simulink model "SVM_Blocks"  (R2021a)
settings: Solver=ode23s  StartTime=0.0  StopTime=.02*20  MaxStep=1e-5  RelTol=1e-3
libraries: spsThreePhaseVIMeasurementLib x5, spsSVPWMGenerator2LevelLib x4, spsThreePhaseSeriesRLCBranchLib x4, spsVoltageMeasurementLib x4, spsDCVoltageSourceLib x3, spsUniversalBridgeLib x3, dsparch4 x2, spsGroundLib x2, spsRMSLib x2, spsAsynchronousMachineSIUnitsLib x1, spsabctoAlphaBetaZeroLib x1, spspowerguiLib x1
settings Model: Creator=Ahmed Mohamed  LastModifiedBy=Ahmed Mohamed
settings DataIOCC: ReturnWorkspaceOutputs=off

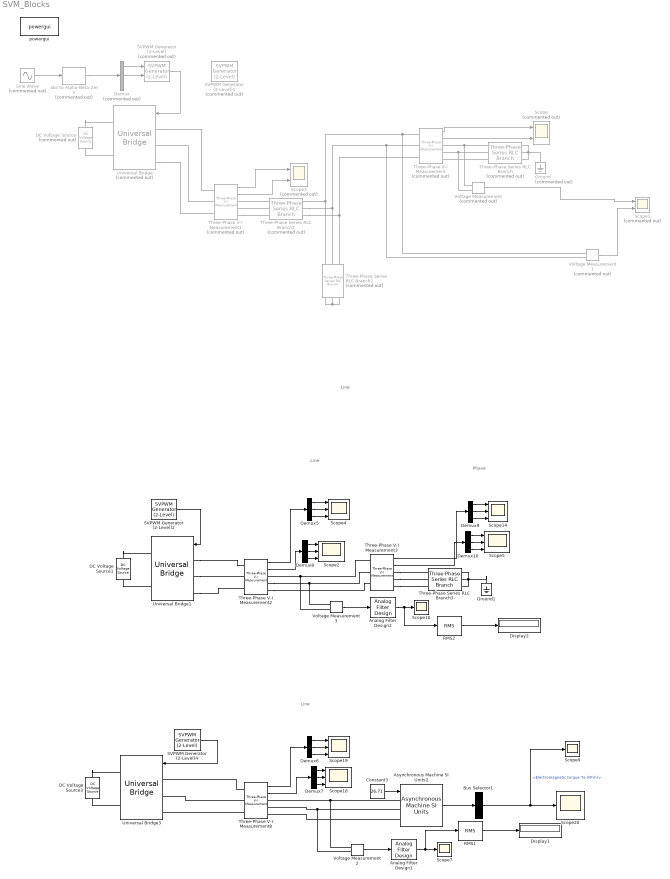
== system SVM_Blocks ==
  note: Line
  note: Phase
  note: Line
  note: Line
  Analog Filter Design1 : dsparch4/Analog Filter Design  method=Butterworth  filttype=Lowpass  N=8  Wlo=2*pi*1000  Whi=80  Rp=2  Rs=40
  Analog Filter Design2 : dsparch4/Analog Filter Design  method=Butterworth  filttype=Lowpass  N=8  Wlo=2*pi*500  Whi=80  Rp=2  Rs=40
  Asynchronous Machine SI Units2 : spsAsynchronousMachineSIUnitsLib/Asynchronous Machine SI Units  RotorType=Squirrel-cage  PresetModel="15:  5.4 HP (4KW)   400 V  50Hz 1430 RPM"  MechanicalLoad=Torque Tm  ShowDetailedParameters=on  ReferenceFrame=Rotor  Units=SI  MeasurementBus=off  NominalParameters=[4000 400 50]  VoltageRatio=1  Stator=[1.405 0.005839]  Rotor=[1.395 0.005839]  Cage1=[0.4155 0.002066]  Cage2=[0.4168 0.0003495]  Lm=0.1722  Mechanical=[0.0131 0.002985 2]  PolePairs=2  InitialConditions=[1 0 0 0 0 0 0 0]  SimulateSaturation=off  Saturation=[14.03593122, 27.81365428, 53.79336849, 72.68890987, 97.98006896, 148.6815601, 215.7428561, 302.9841135, 428.7778367 ; 230, 322, 414, 460, 506, 552, 598, 644, 690]  LoadFlowParameters=1492000  TsPowergui=0  TsBlock=-1  IterativeModel=Trapezoidal non iterative  IterativeDiscreteModel=Trapezoidal non iterative  Pmec=1.492e+006
  Bus Selector1 : BusSelector  OutputSignals=Mechanical.Electromagnetic torque Te (N*m)
  Constant3 : Constant  Value=26.71
  DC Voltage Source : spsDCVoltageSourceLib/DC Voltage Source  Commented=on  Amplitude=540  Measurements=None
  DC Voltage Source1 : spsDCVoltageSourceLib/DC Voltage Source  Amplitude=570  Measurements=None
  DC Voltage Source3 : spsDCVoltageSourceLib/DC Voltage Source  Amplitude=570  Measurements=None
  Demux : Demux  Commented=on  Outputs=3
  Demux{5..10} (6 alike) : Demux  Outputs=3
  Display1 : Display
  Display2 : Display
  Ground : spsGroundLib/Ground  Commented=on  LConnTagsString=a
  Ground1 : spsGroundLib/Ground  LConnTagsString=a
  RMS1 : spsRMSLib/RMS  TrueRMS=off  Freq=50  RMSInit=0  Ts=0
  RMS2 : spsRMSLib/RMS  TrueRMS=off  Freq=50  RMSInit=0  Ts=0
  SVPWM Generator (2-Level) : spsSVPWMGenerator2LevelLib/SVPWM Generator (2-Level)  Commented=on  InputType=alpha-beta components  SwitchingPattern=Pattern #1  Fc=5000  ParUref=[0.8 -30 50]  Ts=0
      settings: SourceProductBaseCode=PS
  SVPWM Generator (2-Level)1 : spsSVPWMGenerator2LevelLib/SVPWM Generator (2-Level)  Commented=on  InputType=Internally generated  SwitchingPattern=Pattern #2  Fc=5000  ParUref=[0.8 -30 50]  Ts=0
      settings: SourceProductBaseCode=PS
  SVPWM Generator (2-Level)2 : spsSVPWMGenerator2LevelLib/SVPWM Generator (2-Level)  InputType=Internally generated  SwitchingPattern=Pattern #1  Fc=10000  ParUref=[1 0 50]  Ts=0
      settings: SourceProductBaseCode=PS
  SVPWM Generator (2-Level)4 : spsSVPWMGenerator2LevelLib/SVPWM Generator (2-Level)  InputType=Internally generated  SwitchingPattern=Pattern #1  Fc=10000  ParUref=[1 0 50]  Ts=0
      settings: SourceProductBaseCode=PS
  Scope : Scope  Commented=on  NumInputPorts=2
  Scope1 : Scope  Commented=on  NumInputPorts=2
  Scope{7,9..10,20} (4 alike) : Scope
  Scope{2,4..5,14,18..19} (6 alike) : Scope  NumInputPorts=3
  Scope3 : Scope  Commented=on  NumInputPorts=2
  Sine Wave : Sin  Commented=on  Amplitude=.99  Frequency=2*50*pi  Phase=[0 -2*pi/3 2*pi/3]  SampleTime=0
  Three-Phase Series RLC Branch : spsThreePhaseSeriesRLCBranchLib/Three-Phase Series RLC Branch  Commented=on  LConnTagsString=A|B|C  RConnTagsString=A|B|C  BranchType=R  Resistance=10  Inductance=1e-3  Capacitance=1e-6  Measurements=None
  Three-Phase Series RLC Branch1 : spsThreePhaseSeriesRLCBranchLib/Three-Phase Series RLC Branch  Commented=on  LConnTagsString=A|B|C  RConnTagsString=A|B|C  BranchType=L  Resistance=10  Inductance=1e-3  Capacitance=1e-6  Measurements=None
  Three-Phase Series RLC Branch2 : spsThreePhaseSeriesRLCBranchLib/Three-Phase Series RLC Branch  Commented=on  LConnTagsString=A|B|C  RConnTagsString=A|B|C  BranchType=C  Resistance=10  Inductance=1e-3  Capacitance=100e-6  Measurements=None
  Three-Phase Series RLC Branch3 : spsThreePhaseSeriesRLCBranchLib/Three-Phase Series RLC Branch  LConnTagsString=A|B|C  RConnTagsString=A|B|C  BranchType=RL  Resistance=7.5*sqrt(2)  Inductance=7.5*sqrt(2)/314  Capacitance=1e-6  Measurements=None
  Three-Phase V-I Measurement : spsThreePhaseVIMeasurementLib/Three-Phase V-I Measurement  Commented=on  VoltageMeasurement=phase-to-ground  SetLabelV=off  LabelV=Vabc  Vpu=off  VpuLL=off  CurrentMeasurement=yes  SetLabelI=off  LabelI=Iabc  Ipu=off  Pbase=100e6  Vbase=500e3  OutputType=Complex  PhasorSimulation=off  PSBequivalent=0
  Three-Phase V-I Measurement1 : spsThreePhaseVIMeasurementLib/Three-Phase V-I Measurement  Commented=on  VoltageMeasurement=phase-to-phase  SetLabelV=off  LabelV=Vabc  Vpu=off  VpuLL=off  CurrentMeasurement=yes  SetLabelI=off  LabelI=Iabc  Ipu=off  Pbase=100e6  Vbase=500e3  OutputType=Complex  PhasorSimulation=off  PSBequivalent=0
  Three-Phase V-I Measurement2 : spsThreePhaseVIMeasurementLib/Three-Phase V-I Measurement  VoltageMeasurement=phase-to-phase  SetLabelV=off  LabelV=Vabc  Vpu=off  VpuLL=off  CurrentMeasurement=yes  SetLabelI=off  LabelI=Iabc  Ipu=off  Pbase=100e6  Vbase=500e3  OutputType=Complex  PhasorSimulation=off  PSBequivalent=0
  Three-Phase V-I Measurement3 : spsThreePhaseVIMeasurementLib/Three-Phase V-I Measurement  VoltageMeasurement=phase-to-ground  SetLabelV=off  LabelV=Vabc  Vpu=off  VpuLL=off  CurrentMeasurement=yes  SetLabelI=off  LabelI=Iabc  Ipu=off  Pbase=100e6  Vbase=500e3  OutputType=Complex  PhasorSimulation=off  PSBequivalent=0
  Three-Phase V-I Measurement8 : spsThreePhaseVIMeasurementLib/Three-Phase V-I Measurement  VoltageMeasurement=phase-to-phase  SetLabelV=off  LabelV=Vabc  Vpu=off  VpuLL=off  CurrentMeasurement=yes  SetLabelI=off  LabelI=Iabc  Ipu=off  Pbase=100e6  Vbase=500e3  OutputType=Complex  PhasorSimulation=off  PSBequivalent=0
  Universal Bridge : spsUniversalBridgeLib/Universal Bridge  Commented=on  Arms=3  SnubberResistance=1e5  SnubberCapacitance=inf  Device=IGBT / Diodes  Ron=1e-3  Lon=0  ForwardVoltages="[  0  0  ]"  ForwardVoltage=0  GTOparameters=[ 10e-6 , 20e-6 ]  IGBTparameters=[ 1e-6 , 2e-6 ]  Measurements=None  Measurements_2=None  converterType=Rectifier
  Universal Bridge1 : spsUniversalBridgeLib/Universal Bridge  Arms=3  SnubberResistance=1e5  SnubberCapacitance=inf  Device=IGBT / Diodes  Ron=1e-3  Lon=0  ForwardVoltages="[  0  0  ]"  ForwardVoltage=0  GTOparameters=[ 10e-6 , 20e-6 ]  IGBTparameters=[ 1e-6 , 2e-6 ]  Measurements=None  Measurements_2=None  converterType=Rectifier
  Universal Bridge3 : spsUniversalBridgeLib/Universal Bridge  Arms=3  SnubberResistance=1e5  SnubberCapacitance=inf  Device=IGBT / Diodes  Ron=1e-3  Lon=0  ForwardVoltages="[  0  0  ]"  ForwardVoltage=0  GTOparameters=[ 10e-6 , 20e-6 ]  IGBTparameters=[ 1e-6 , 2e-6 ]  Measurements=None  Measurements_2=None  converterType=Rectifier
  Voltage Measurement : spsVoltageMeasurementLib/Voltage Measurement  Commented=on  PhasorSimulation=off  OutputType=Complex  PSBequivalent=0
  Voltage Measurement1 : spsVoltageMeasurementLib/Voltage Measurement  Commented=on  PhasorSimulation=off  OutputType=Complex  PSBequivalent=0
  Voltage Measurement2 : spsVoltageMeasurementLib/Voltage Measurement  PhasorSimulation=off  OutputType=Complex  PSBequivalent=0
  Voltage Measurement3 : spsVoltageMeasurementLib/Voltage Measurement  PhasorSimulation=off  OutputType=Complex  PSBequivalent=0
  abc to Alpha-Beta-Zero : spsabctoAlphaBetaZeroLib/abc to Alpha-Beta-Zero  Commented=on
      settings: SourceProductBaseCode=PS
  powergui : spspowerguiLib/powergui  Priority=1  SimulationMode=Continuous  SampleTime=50e-6  frequency=60  Iterations=50  frequencyindice=0  Pbase=100e6  ErrMax=1e-4  UnitsV=kV  UnitsW=MW  buscounter=0  FunctionMessages=off  echomessages=off  EnableUseOfTLC=off  CurrentSourceSwitches=off  DisableSnubberDevices=off  DisableRonSwitches=off  DisableVfSwitches=off  DisplayEquations=off  AutomaticDiscreteSolvers=off  SolverType=Tustin/Backward Euler (TBE)  Interpol=off  ExternalGateDelay=off  methode=off  Ts=100  x0status=blocks  SPID=on  SwTol=0  HookPort=off  NonlinearTolerance=1e-4  nMaxIteration=100  ContinueOnMaxIteration=off  RestoreLinks=warning  ResistiveCurrentMeasurement=off  Frange=[0:2:500]  Ylog=off  Xlog=on  ShowGrid=off  save=off  variable=ZData  structure=0  ZoomFFT=off  StartTime=0.0  cycles=1  DisplayStyle=1  fundamental=60  FreqAxis=off  MaxFrequency=1000  frequencyindicesteady=1  RmsSteady=1  display=off
  wires:
  Sine Wave/1 -> abc to Alpha-Beta-Zero/1
  abc to Alpha-Beta-Zero/1 -> Demux/1
  Demux/1 -> SVPWM Generator (2-Level)/1
  Demux/2 -> SVPWM Generator (2-Level)/2
  SVPWM Generator (2-Level)/1 -> Universal Bridge/1
  Three-Phase V-I Measurement/1 -> Scope/1
  Three-Phase V-I Measurement/2 -> Scope/2
  Voltage Measurement/1 -> Scope1/1
  Three-Phase V-I Measurement1/1 -> Scope3/1
  Three-Phase V-I Measurement1/2 -> Scope3/2
  Voltage Measurement1/1 -> Scope1/2
  SVPWM Generator (2-Level)2/1 -> Universal Bridge1/1
  Demux10/1 -> Scope5/1
  Demux5/1 -> Scope4/1
  Demux5/3 -> Scope4/3
  Demux10/3 -> Scope5/3
  Demux9/3 -> Scope14/3
  Three-Phase V-I Measurement3/2 -> Demux10/1
  Three-Phase V-I Measurement3/1 -> Demux9/1
  Demux5/2 -> Scope4/2
  Demux10/2 -> Scope5/2
  Demux8/1 -> Scope2/1
  Demux9/2 -> Scope14/2
  Three-Phase V-I Measurement2/2 -> Demux8/1
  Demux8/2 -> Scope2/2
  Three-Phase V-I Measurement2/1 -> Demux5/1
  Demux9/1 -> Scope14/1
  Demux8/3 -> Scope2/3
  SVPWM Generator (2-Level)4/1 -> Universal Bridge3/1
  Three-Phase V-I Measurement8/1 -> Demux6/1
  Asynchronous Machine SI Units2/1 -> Bus Selector1/1
  Three-Phase V-I Measurement8/2 -> Demux7/1
  Bus Selector1/1 -> Scope9/1, Scope20/1  "<Electromagnetic torque Te (N*m)>"
  Demux7/3 -> Scope18/3
  Demux7/2 -> Scope18/2
  Demux6/1 -> Scope19/1
  Demux7/1 -> Scope18/1
  Demux6/3 -> Scope19/3
  Constant3/1 -> Asynchronous Machine SI Units2/1
  Demux6/2 -> Scope19/2
  RMS1/1 -> Display1/1
  Analog Filter Design1/1 -> Scope7/1, RMS1/1
  Voltage Measurement2/1 -> Analog Filter Design1/1
  Voltage Measurement3/1 -> Analog Filter Design2/1
  Analog Filter Design2/1 -> Scope10/1, RMS2/1
  RMS2/1 -> Display2/1
  connections:
  DC Voltage Source/RConn1 -- Universal Bridge/RConn1
  DC Voltage Source/LConn1 -- Universal Bridge/RConn2
  Three-Phase V-I Measurement1/LConn2 -- Universal Bridge/LConn2
  Universal Bridge/LConn1 -- Three-Phase V-I Measurement1/LConn1
  Universal Bridge/LConn3 -- Three-Phase V-I Measurement1/LConn3
  Three-Phase Series RLC Branch/LConn1 -- Voltage Measurement/LConn1 -- Three-Phase V-I Measurement/RConn1
  Three-Phase Series RLC Branch/LConn2 -- Voltage Measurement/LConn2 -- Three-Phase V-I Measurement/RConn2
  Three-Phase Series RLC Branch/LConn3 -- Three-Phase V-I Measurement/RConn3
  Three-Phase Series RLC Branch/RConn1 -- Ground/LConn1 -- Three-Phase Series RLC Branch/RConn2 -- Three-Phase Series RLC Branch/RConn3
  Three-Phase Series RLC Branch1/LConn1 -- Three-Phase V-I Measurement1/RConn1
  Three-Phase Series RLC Branch1/LConn2 -- Three-Phase V-I Measurement1/RConn2
  Three-Phase Series RLC Branch1/RConn1 -- Voltage Measurement1/LConn1 -- Three-Phase V-I Measurement/LConn1 -- Three-Phase Series RLC Branch2/LConn1
  Three-Phase Series RLC Branch1/RConn2 -- Voltage Measurement1/LConn2 -- Three-Phase V-I Measurement/LConn2 -- Three-Phase Series RLC Branch2/LConn2
  Three-Phase Series RLC Branch1/RConn3 -- Three-Phase V-I Measurement/LConn3 -- Three-Phase Series RLC Branch2/LConn3
  Three-Phase Series RLC Branch2/RConn1 -- Three-Phase Series RLC Branch2/RConn2 -- Three-Phase Series RLC Branch2/RConn3
  Three-Phase V-I Measurement1/RConn3 -- Three-Phase Series RLC Branch1/LConn3
  DC Voltage Source1/RConn1 -- Universal Bridge1/RConn1
  DC Voltage Source1/LConn1 -- Universal Bridge1/RConn2
  Three-Phase Series RLC Branch3/RConn2 -- Three-Phase Series RLC Branch3/RConn3 -- Three-Phase Series RLC Branch3/RConn1 -- Ground1/LConn1
  Three-Phase V-I Measurement3/RConn3 -- Three-Phase Series RLC Branch3/LConn3
  Three-Phase V-I Measurement3/RConn2 -- Three-Phase Series RLC Branch3/LConn2
  Three-Phase V-I Measurement2/RConn3 -- Three-Phase V-I Measurement3/LConn3
  Three-Phase V-I Measurement3/LConn1 -- Voltage Measurement3/LConn2 -- Three-Phase V-I Measurement2/RConn1
  Three-Phase V-I Measurement2/RConn2 -- Voltage Measurement3/LConn1 -- Three-Phase V-I Measurement3/LConn2
  Three-Phase V-I Measurement3/RConn1 -- Three-Phase Series RLC Branch3/LConn1
  Universal Bridge1/LConn1 -- Three-Phase V-I Measurement2/LConn1
  Universal Bridge1/LConn2 -- Three-Phase V-I Measurement2/LConn2
  Universal Bridge1/LConn3 -- Three-Phase V-I Measurement2/LConn3
  Three-Phase V-I Measurement8/LConn3 -- Universal Bridge3/LConn3
  Three-Phase V-I Measurement8/LConn1 -- Universal Bridge3/LConn1
  Three-Phase V-I Measurement8/LConn2 -- Universal Bridge3/LConn2
  DC Voltage Source3/LConn1 -- Universal Bridge3/RConn2
  DC Voltage Source3/RConn1 -- Universal Bridge3/RConn1
  Asynchronous Machine SI Units2/LConn3 -- Three-Phase V-I Measurement8/RConn3
  Asynchronous Machine SI Units2/LConn1 -- Voltage Measurement2/LConn1 -- Three-Phase V-I Measurement8/RConn1
  Asynchronous Machine SI Units2/LConn2 -- Voltage Measurement2/LConn2 -- Three-Phase V-I Measurement8/RConn2
